simulink model "Elevator_project"  (R2020a)
settings: Solver=FixedStepAuto  StartTime=0.0  StopTime=inf  FixedStep=0.1  RelTol=1e-3
settings Model: EnablePacing=on  Creator=jatin  LastModifiedBy=jatin
settings RTWCC: GenCodeOnly=on  PackageGeneratedCodeAndArtifacts=on
settings GRTTargetCC: MatFileLogging=off
settings ConfigComp: DVMode=PropertyProving  DVMaxProcessTime=NaN  DVTestSuiteOptimization=Auto  DVDetectOutOfBounds=on

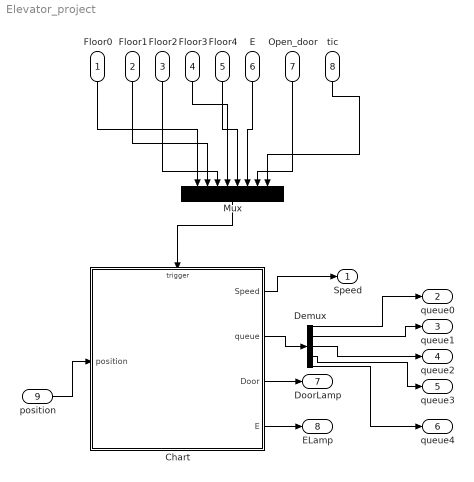
== system Elevator_project ==
  Floor0 : Inport
  Floor1 : Inport  Port=2
  Floor2 : Inport  Port=3
  Floor3 : Inport  Port=4
  Floor4 : Inport  Port=5
  E : Inport  Port=6
  Open_door : Inport  Port=7
  tic : Inport  Port=8
  position : Inport  Port=9
  Chart : Stateflow chart  TreatAsAtomicUnit=on
  Demux : Demux  Outputs=5
  Mux : Mux  Inputs=8
  Speed : Outport
  queue0 : Outport  Port=2
  queue1 : Outport  Port=3
  queue2 : Outport  Port=4
  queue3 : Outport  Port=5
  queue4 : Outport  Port=6
  DoorLamp : Outport  Port=7
  ELamp : Outport  Port=8
  wires:
  Mux/1 -> Chart/Trigger
  Chart/1(Speed) -> Speed/1
  Chart/2(queue) -> Demux/1
  Chart/3(Door) -> DoorLamp/1
  Floor0/1 -> Mux/1
  Floor1/1 -> Mux/2
  Floor2/1 -> Mux/3
  Floor3/1 -> Mux/4
  Floor4/1 -> Mux/5
  E/1 -> Mux/6
  Open_door/1 -> Mux/7
  tic/1 -> Mux/8
  Demux/2 -> queue1/1
  Demux/1 -> queue0/1
  Demux/3 -> queue2/1
  Demux/4 -> queue3/1
  Demux/5 -> queue4/1
  Chart/4(E) -> ELamp/1
  position/1 -> Chart/1(position)

== stateflow chart Elevator_project/Chart ==
  settings: executeAtInitialization=1
  state Init
    on floor0: queue(1)=1;
    on floor1: queue(2)=1;
    on floor2: queue(3)=1;
    on floor3: queue(4)=1;
    on floor4: queue(5)=1;
    on Open_doors: open_door=1;
    du: Error_check();
    state Up
      Speed=0.2;
      dir=1;
      floor_check();
    state Door
      Door=1;queue(dest)=0;
    state Idle_state
    state Emergency
      Speed=0;
    state Down
      Speed=-0.2;
      dir=-1;
      floor_check();
    Idle_state -> Door [order 2] : [current_floor()==1 || (open_door==1 && Speed==0)]{open_door=0;}
    Up -> Door [order 2] : [position>=dest-1]{Speed=0;}
    Idle_state -> Up [order 3] : [floor_check==1]
    Up -> Emergency [order 1] : Emergency{u=1;E=1;}
    Emergency -> Up [order 2] : Emergency[u==1]{u=0;E=0;}
    Door -> Door [order 2] : [open_door==1]{open_door=0;}
    (default) -> Idle_state
    Door -> Emergency [order 1] : Emergency{do=1;E=1;}
    Idle_state -> Emergency [order 1] : Emergency{i=1;E=1;}
    Emergency -> Door [order 3] : Emergency[do==1]{do=0;E=0;}
    Emergency -> Idle_state [order 1] : Emergency[i==1]{E=0;i=0;}
    Down -> Door [order 1] : [position<=dest-0.98]{Speed=0;}
    Door -> Idle_state [order 3] : [after(5,tic)]{Door=0;}
    Down -> Emergency [order 2] : Emergency{d=1;E=1;}
    Emergency -> Down [order 4] : Emergency[d==1]{d=0;E=0;}
    Idle_state -> Down [order 4] : [floor_check==0]
  (default) -> Init : {open_door=0;dest=1;Speed=0;queue(1)=0;E=0;dir=0;i=0;u=0;d=0;do=0;}
  data: out function_output; o function_output; Speed output; dest local; queue output double size=[1 5]; Door output; E output; d local; do local; i local; u local; dir local; open_door local; position input
  events: floor0 input RISING_EDGE_EVENT; floor1 input RISING_EDGE_EVENT; floor2 input RISING_EDGE_EVENT; floor3 input RISING_EDGE_EVENT; floor4 input RISING_EDGE_EVENT; Emergency input RISING_EDGE_EVENT; Open_doors input RISING_EDGE_EVENT; tic input RISING_EDGE_EVENT
  function out = floor_check:
    | function out = floor_check
    | if dir>0
    |     if queue(2)&& position<1
    |         dest=2;
    |         out=1;  
    |     elseif queue(3) && position<2
    |         dest=3;
    |         out=1;
    |     elseif queue(4)&& position<3
    |         dest=4;
    |         out=1;
    |     elseif queue(5) && position~=4
    |         dest=5;
    |         out=1;
    |     else
    |         dir=0;
    |         out=-1;
    |     end
    | elseif dir<0
    |     if queue(4)&& position>3
    |         dest=4;
    |         out=0;    
    |     elseif queue(3)&& position>2
    |         dest=3;
    |         out=0;
    |     elseif queue(2)&& position>1
    |         dest=2;
    |         out=0;
    |     elseif queue(1)&& position~=0
    |         dest=1;
    |         out=0;
    |     else
    |         dir=0;
    |         out=-1;
    |     end
    | else
    |     if queue(1) && position~=0
    |         dest=1;
    |         out=0;
    |     elseif queue(2)
    |         if position>1
    |             dest=2;
    |             out=0;
    |         elseif position<1
    |             dest=2;
    |             out=1;
    |         else out=-1;
    |             dir=0;
    |         end
    |     elseif queue(3)
    |         if position>2
    |             dest=3;
    |             out=0;
    |         elseif position<2
    |             dest=3;
    |             out=1;
    |         else
    |             out=-1;
    |             dir=0;
    |         end
    |     elseif queue(4)
    |         if position>3
    |             dest=4;
    |             out=0;
    |         elseif position<3
    |             dest=4;
    |             out=1;
    |         else
    |             out=-1;
    |             dir=0;
    |         end
    |     elseif queue(5) && position~=4
    |         dest=5;
    |         out=1;
    |     else
    |         out=-1;
    |         dir=0;
    |     end
    | end
  function Error_check:
    | function Error_check
    | cur_pos=position;
    | if position>4.1 && position<0
    |     Speed=0;
    | elseif (position==cur_pos + 0.5) || (position == cur_pos - 0.5)
    |      Speed=0;
    | elseif (Speed>0 || Speed<0) && Door==1
    |     Speed=0;
    |     Door=0;
    | end
  function o=current_floor:
    | function o=current_floor
    | if dir==0
    |     if queue(1) && queue(2)==0 && queue(3)==0 && queue(4)==0 && queue(5)==0 && position<1 && position>=0
    |         o=1;
    |         dest=1;
    |     elseif queue(1)==0 && queue(2) && queue(3)==0 && queue(4)==0 && queue(5)==0 && position<2 && position>=1
    |         o=1;
    |         dest=2;
    |     elseif queue(1)==0 && queue(2)==0 && queue(3) && queue(4)==0 && queue(5)==0 && position<3 && position>=2
    |         o=1;
    |         dest=3;
    |     elseif queue(1)==0 && queue(2)==0 && queue(3)==0 && queue(4) && queue(5)==0 && position<4 && position>=3
    |         o=1;
    |         dest=4;
    |     elseif queue(1)==0 && queue(2)==0 && queue(3)==0 && queue(4)==0 && queue(5) && position>=4
    |         o=1;
    |         dest=5;
    |     else
    |         o=0;
    |     end
    | else
    |     o=0;
    | end
